simulink model "HybridModel"  (R2020a)
settings: Solver=FixedStepAuto  StartTime=0  StopTime=10.67  FixedStep=0.01  RelTol=1e-3
undefined symbols (not defined in the file): delay, VSA
libraries: cstblocks x1
settings Model: Creator=Brock  LastModifiedBy=Brock

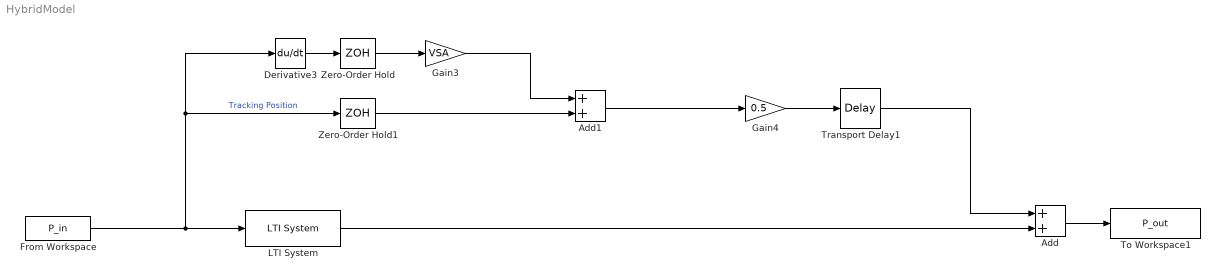
== system HybridModel ==
  Add : Sum
  Add1 : Sum
  Derivative3 : Derivative
  From Workspace : FromWorkspace  VariableName=P_in
  Gain3 : Gain  Gain=VSA
  Gain4 : Gain  Gain=0.5
  LTI System : cstblocks/LTI System  sys=TF_sm  IC=[]
  To Workspace1 : ToWorkspace  VariableName=P_out  SampleTime=-1
  Transport Delay1 : TransportDelay  DelayTime=delay
  Zero-Order Hold : ZeroOrderHold  SampleTime=0.1
  Zero-Order Hold1 : ZeroOrderHold  SampleTime=0.1
  wires:
  From Workspace/1 -> LTI System/1, Zero-Order Hold1/1, Derivative3/1  "Tracking Position"
  Add/1 -> To Workspace1/1
  Derivative3/1 -> Zero-Order Hold/1
  Zero-Order Hold/1 -> Gain3/1
  Gain3/1 -> Add1/1
  Zero-Order Hold1/1 -> Add1/2
  Add1/1 -> Gain4/1
  Gain4/1 -> Transport Delay1/1
  Transport Delay1/1 -> Add/1
  LTI System/1 -> Add/2
